simulink model "Modell_13_1_v2"  (R2018a)
settings: Solver=VariableStepAuto  StartTime=0.0  StopTime=10  MaxStep=0.001  RelTol=1e-3
InitFcn:
  | init_13_1_v2
values from neighbouring files (symbols this model uses):
  a = 1    [init_13_1.m]    (also in init_13_1_v2.m; init_13_4.m)
  b = 1    [init.m]    (also in init_13_1.m; init_13_1_v2.m = 0.1111; init_13_4.m)
  c = 0.5    [init.m]    (also in init_13_1.m; init_13_1_v2.m = 0.8333; init_13_4.m = 1)
  grenze = 20    [init_13_1_v2.m]
  grenzeSalz = 30    [init_13_1_v2.m]
  kS = 1    [init_13_1_v2.m]    (also in init_13_4.m = 0.3)
  kT = 1    [init_13_1_v2.m]    (also in init_13_4.m)
  kw = 0.1    [init_13_1_v2.m]
  kwS = 0.35    [init_13_1_v2.m]
  S01 = 30    [init_13_1_v2.m]    (also in init_13_4.m = 1.7)
  S02 = 35    [init_13_1_v2.m]    (also in init_13_4.m = 0.5)
  S1 = 31.87    [init_13_1_v2.m]
  S2 = 33.13    [init_13_1_v2.m]
  T01 = 29    [init_13_1_v2.m]    (also in init_13_4.m = 1.9)
  T02 = 12    [init_13_1_v2.m]    (also in init_13_4.m = 0.8)
  T1 = 10.8    [init_13_1_v2.m]
  T2 = 9.2    [init_13_1_v2.m]
libraries: simulink x2
settings Model: Creator=Uni  LastModifiedBy=Uni

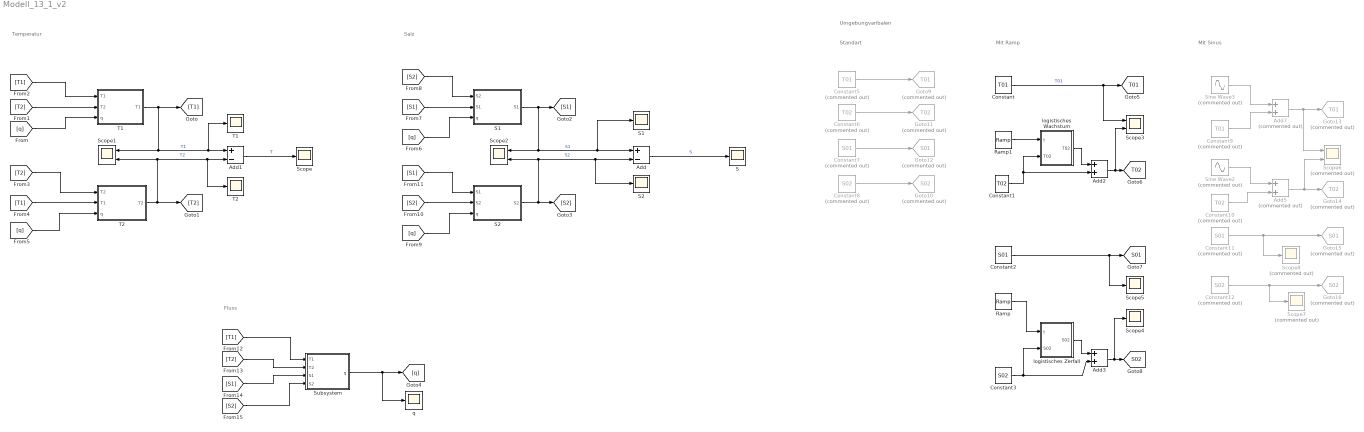
== system Modell_13_1_v2 ==
  note: Temperatur
  note: Salz
  note: Fluss
  note: Umgebungvaribalen
  note: Standart
  note: Mit Ramp
  note: Mit Sinus
  Add : Sum  Inputs=+-
  Add1 : Sum  Inputs=+-
  Add2 : Sum
  Add3 : Sum
  Add5 : Sum  Commented=on
  Add7 : Sum  Commented=on
  Constant : Constant  Value=T01
  Constant1 : Constant  Value=T02
  Constant10 : Constant  Commented=on  Value=T02
  Constant11 : Constant  Commented=on  Value=S01
  Constant12 : Constant  Commented=on  Value=S02
  Constant2 : Constant  Value=S01
  Constant3 : Constant  Value=S02
  Constant5 : Constant  Commented=on  Value=T01
  Constant6 : Constant  Commented=on  Value=T02
  Constant7 : Constant  Commented=on  Value=S01
  Constant8 : Constant  Commented=on  Value=S02
  Constant9 : Constant  Commented=on  Value=T01
  Goto10 : Goto  Commented=on  GotoTag=S02  TagVisibility=global
  Goto11 : Goto  Commented=on  GotoTag=T02  TagVisibility=global
  Goto12 : Goto  Commented=on  GotoTag=S01  TagVisibility=global
  Goto13 : Goto  Commented=on  GotoTag=T01  TagVisibility=global
  Goto14 : Goto  Commented=on  GotoTag=T02  TagVisibility=global
  Goto15 : Goto  Commented=on  GotoTag=S01  TagVisibility=global
  Goto16 : Goto  Commented=on  GotoTag=S02  TagVisibility=global
  Goto9 : Goto  Commented=on  GotoTag=T01  TagVisibility=global
  Ramp : simulink/Sources/Ramp  slope=1  start=0  InitialOutput=0
  Ramp1 : simulink/Sources/Ramp  slope=1  start=0  InitialOutput=0
  S : Scope
  S1 : Scope
  "S1 " : Subsystem
  S2 : Scope
  "S2 " : Subsystem
  Scope : Scope
  Scope1 : Scope  NumInputPorts=2
  Scope2 : Scope  NumInputPorts=2
  Scope3 : Scope  NumInputPorts=2
  Scope4 : Scope
  Scope5 : Scope
  Scope6 : Scope  Commented=on  NumInputPorts=2
  Scope7 : Scope  Commented=on
  Scope8 : Scope  Commented=on
  Sine Wave2 : Sin  Commented=on  Amplitude=7  Frequency=2*pi  Phase=pi/2  SampleTime=0
  Sine Wave3 : Sin  Commented=on  Amplitude=4  Frequency=2*pi  Phase=pi/2  SampleTime=0
  Subsystem : Subsystem
  T1 : Subsystem
  "T1 " : Scope
  T2 : Subsystem
  "T2 " : Scope
  logistisches Wachstum : Subsystem
  logistisches Zerfall : Subsystem
  q : Scope
  tag scope: S01=global, S02=global, T01=global, T02=global
  wires:
  [T1] -> T1/1("T1 ")
  [T2] -> T1/2("T2 ")
  [q] -> T1/3("q ")
  T1/1(T1) -> Scope1/1, "T1 "/1, Add1/1, [T1]  "T1"
  T2/1("T2 ") -> [T2], Scope1/2, "T2 "/1, Add1/2  "T2"
  [T2] -> T2/1("T2 ")
  [T1] -> T2/2(T1)
  [q] -> T2/3("q ")
  [S2] -> "S1 "/1(S2)
  [S1] -> "S1 "/2("S1 ")
  [q] -> "S1 "/3(q)
  "S1 "/1(S1) -> Scope2/1, S1/1, Add/1, [S1]  "S1"
  [q] -> "S2 "/3(q)
  "S2 "/1(S2) -> [S2], Scope2/2, S2/1, Add/2  "S2"
  [S2] -> "S2 "/2("S2 ")
  [S1] -> "S2 "/1("S1 ")
  [T1] -> Subsystem/1(T1)
  [T2] -> Subsystem/2(T2)
  [S1] -> Subsystem/3(S1)
  [S2] -> Subsystem/4(S2)
  Subsystem/1(q) -> q/1, [q]
  Add/1 -> S/1  "S"
  Add1/1 -> Scope/1  "T"
  Constant2/1 -> Scope5/1, [S01]
  Add3/1 -> Scope4/1, [S02]
  Constant5/1 -> Goto9/1
  Constant8/1 -> Goto10/1
  Constant6/1 -> Goto11/1
  Constant7/1 -> Goto12/1
  Add7/1 -> Scope6/1, Goto13/1
  Constant9/1 -> Add7/2
  Constant10/1 -> Add5/2
  Constant11/1 -> Scope8/1, Goto15/1
  Add5/1 -> Scope6/2, Goto14/1
  Sine Wave3/1 -> Add7/1
  Sine Wave2/1 -> Add5/1
  Constant12/1 -> Scope7/1, Goto16/1
  Constant/1 -> Scope3/1, [T01]  "T01"
  Ramp1/1 -> logistisches Wachstum/1(t)
  Constant1/1 -> Add2/2, logistisches Wachstum/2("T02 ")
  logistisches Wachstum/1(T02) -> Add2/1
  Add2/1 -> Scope3/2, [T02]
  logistisches Zerfall/1(S02) -> Add3/1
  Constant3/1 -> Add3/2, logistisches Zerfall/2("S02 ")
  Ramp/1 -> logistisches Zerfall/1(t)

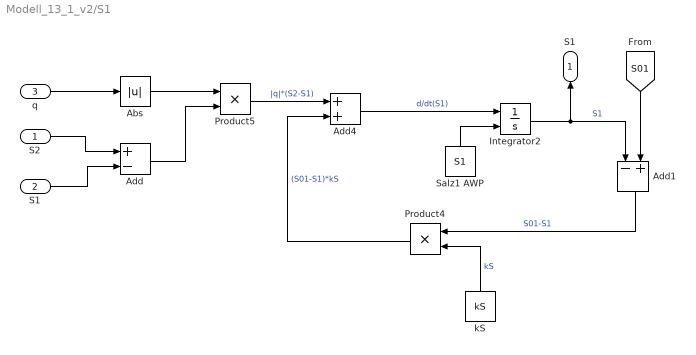
== system Modell_13_1_v2/S1  ==
  S2 : Inport
  "S1 " : Inport  Port=2
  q : Inport  Port=3
  Abs : Abs
  Add : Sum  Inputs=+-
  Add1 : Sum  Inputs=-+
  Add4 : Sum
  Integrator2 : Integrator  InitialConditionSource=external
  Product4 : Product
  Product5 : Product
  Salz1 AWP : Constant  Value=S1
  kS : Constant  Value=kS
  S1 : Outport
  wires:
  q/1 -> Abs/1
  Product4/1 -> Add4/2  "(S01-S1)*kS"
  Integrator2/1 -> Add1/1, S1/1  "S1"
  Add4/1 -> Integrator2/1  "d/dt(S1)"
  Product5/1 -> Add4/1  "|q|*(S2-S1)"
  Add/1 -> Product5/2
  Add1/1 -> Product4/1  "S01-S1"
  [S01] -> Add1/2
  S2/1 -> Add/1
  Salz1 AWP/1 -> Integrator2/2
  kS/1 -> Product4/2  "kS"
  "S1 "/1 -> Add/2
  Abs/1 -> Product5/1

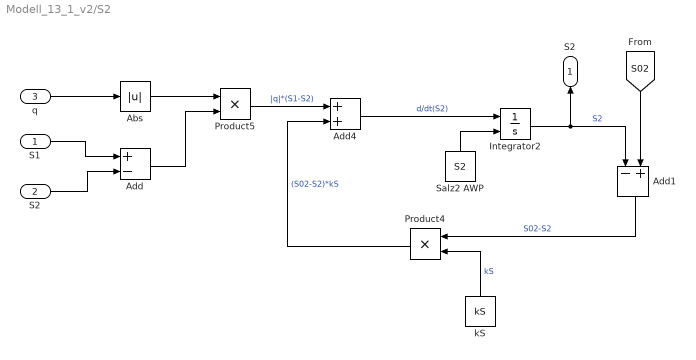
== system Modell_13_1_v2/S2  ==
  "S1 " : Inport
  "S2 " : Inport  Port=2
  q : Inport  Port=3
  Abs : Abs
  Add : Sum  Inputs=+-
  Add1 : Sum  Inputs=-+
  Add4 : Sum
  Integrator2 : Integrator  InitialConditionSource=external
  Product4 : Product
  Product5 : Product
  Salz2 AWP : Constant  Value=S2
  kS : Constant  Value=kS
  S2 : Outport
  wires:
  q/1 -> Abs/1
  Product4/1 -> Add4/2  "(S02-S2)*kS"
  Integrator2/1 -> Add1/1, S2/1  "S2"
  Add4/1 -> Integrator2/1  "d/dt(S2)"
  Product5/1 -> Add4/1  "|q|*(S1-S2)"
  Add/1 -> Product5/2
  Add1/1 -> Product4/1  "S02-S2"
  "S1 "/1 -> Add/1
  Salz2 AWP/1 -> Integrator2/2
  kS/1 -> Product4/2  "kS"
  "S2 "/1 -> Add/2
  Abs/1 -> Product5/1
  [S02] -> Add1/2

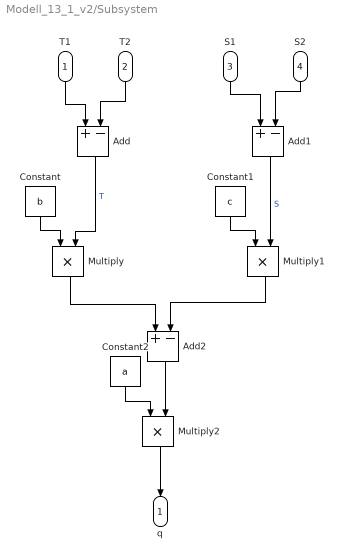
== system Modell_13_1_v2/Subsystem ==
  T1 : Inport
  T2 : Inport  Port=2
  S1 : Inport  Port=3
  S2 : Inport  Port=4
  Add : Sum  Inputs=+-
  Add1 : Sum  Inputs=+-
  Add2 : Sum  Inputs=+-
  Constant : Constant  Value=b
  Constant1 : Constant  Value=c
  Constant2 : Constant  Value=a
  Multiply : Product
  Multiply1 : Product
  Multiply2 : Product
  q : Outport
  wires:
  Add/1 -> Multiply/2  "T"
  Constant2/1 -> Multiply2/1
  Add1/1 -> Multiply1/2  "S"
  Constant1/1 -> Multiply1/1
  Multiply2/1 -> q/1
  Multiply/1 -> Add2/1
  Add2/1 -> Multiply2/2
  Multiply1/1 -> Add2/2
  Constant/1 -> Multiply/1
  T1/1 -> Add/1
  T2/1 -> Add/2
  S2/1 -> Add1/2
  S1/1 -> Add1/1

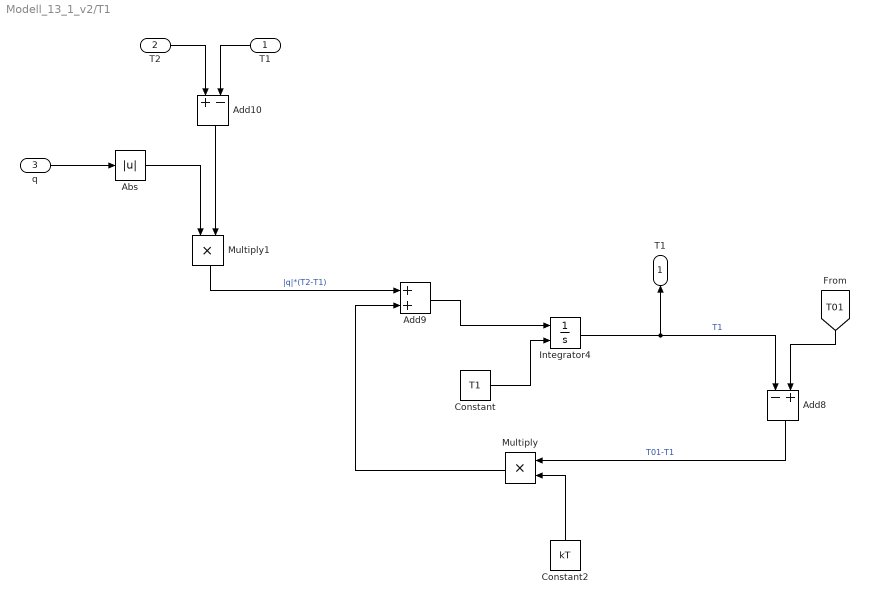
== system Modell_13_1_v2/T1 ==
  "T1 " : Inport
  "T2 " : Inport  Port=2
  "q " : Inport  Port=3
  Abs : Abs
  Add10 : Sum  Inputs=+-
  Add8 : Sum  Inputs=-+
  Add9 : Sum
  Constant : Constant  Value=T1
  Constant2 : Constant  Value=kT
  Integrator4 : Integrator  InitialConditionSource=external
  Multiply : Product
  Multiply1 : Product
  T1 : Outport
  wires:
  Add8/1 -> Multiply/1  "T01-T1"
  Multiply1/1 -> Add9/1  "|q|*(T2-T1)"
  Constant2/1 -> Multiply/2
  Add10/1 -> Multiply1/2
  "q "/1 -> Abs/1
  Constant/1 -> Integrator4/2
  Multiply/1 -> Add9/2
  Integrator4/1 -> Add8/1, T1/1  "T1"
  Add9/1 -> Integrator4/1
  [T01] -> Add8/2
  "T1 "/1 -> Add10/2
  "T2 "/1 -> Add10/1
  Abs/1 -> Multiply1/1

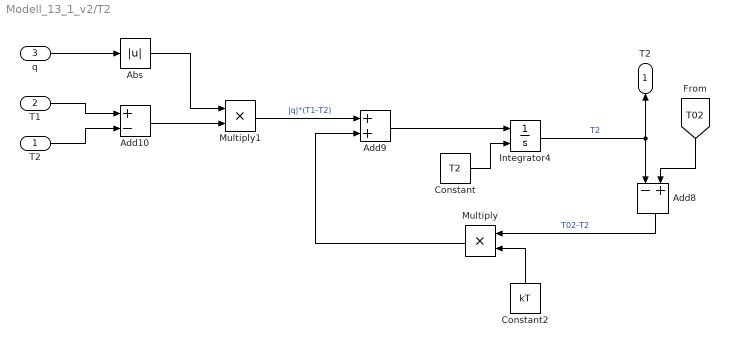
== system Modell_13_1_v2/T2 ==
  "T2 " : Inport
  T1 : Inport  Port=2
  "q " : Inport  Port=3
  Abs : Abs
  Add10 : Sum  Inputs=+-
  Add8 : Sum  Inputs=-+
  Add9 : Sum
  Constant : Constant  Value=T2
  Constant2 : Constant  Value=kT
  Integrator4 : Integrator  InitialConditionSource=external
  Multiply : Product
  Multiply1 : Product
  "T2 " : Outport
  wires:
  Add8/1 -> Multiply/1  "T02-T2"
  Multiply1/1 -> Add9/1  "|q|*(T1-T2)"
  Constant2/1 -> Multiply/2
  Add10/1 -> Multiply1/2
  "q "/1 -> Abs/1
  Constant/1 -> Integrator4/2
  Multiply/1 -> Add9/2
  Integrator4/1 -> Add8/1, "T2 "/1  "T2"
  Add9/1 -> Integrator4/1
  [T02] -> Add8/2
  "T2 "/1 -> Add10/2
  T1/1 -> Add10/1
  Abs/1 -> Multiply1/1

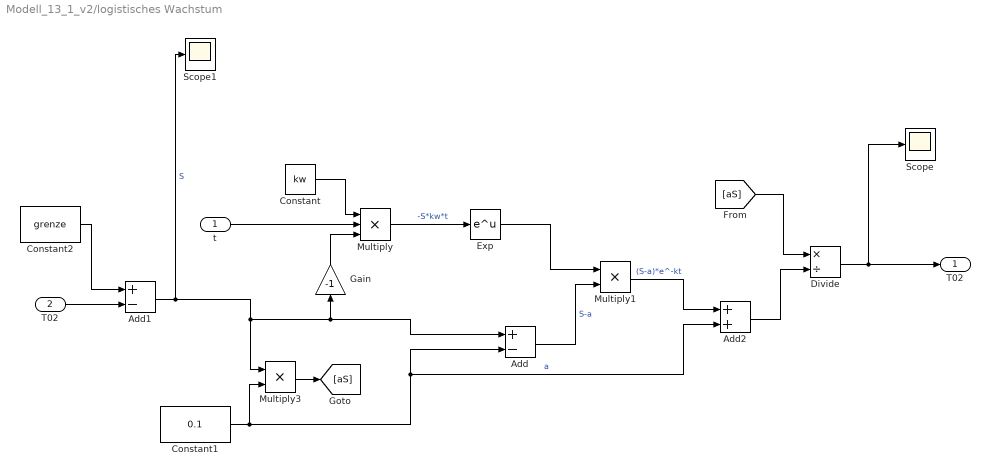
== system Modell_13_1_v2/logistisches Wachstum ==
  t : Inport
  "T02 " : Inport  Port=2
  Add : Sum  Inputs=+-
  Add1 : Sum  Inputs=+-
  Add2 : Sum
  Constant : Constant  Value=kw
  Constant1 : Constant  Value=0.1
  Constant2 : Constant  Value=grenze
  Divide : Product  Inputs=*/
  Exp : Math  SaturateOnIntegerOverflow=on
  Gain : Gain  Gain=-1
  Multiply : Product  Inputs=3
  Multiply1 : Product
  Multiply3 : Product
  Scope : Scope
  Scope1 : Scope
  T02 : Outport
  wires:
  Constant/1 -> Multiply/1
  t/1 -> Multiply/2
  Multiply/1 -> Exp/1  "-S*kw*t"
  Exp/1 -> Multiply1/1
  Multiply1/1 -> Add2/1  "(S-a)*e^-kt"
  Divide/1 -> Scope/1, T02/1
  Add/1 -> Multiply1/2  "S-a"
  Constant1/1 -> Multiply3/2, Add/2, Add2/2  "a"
  Add1/1 -> Scope1/1, Add/1, Gain/1, Multiply3/1  "S"
  Gain/1 -> Multiply/3
  Multiply3/1 -> [aS]
  Add2/1 -> Divide/2
  [aS] -> Divide/1
  Constant2/1 -> Add1/1
  "T02 "/1 -> Add1/2

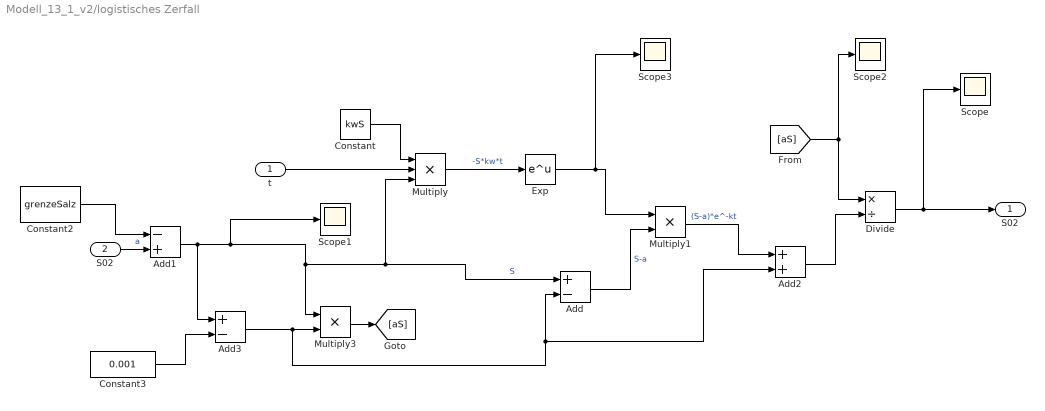
== system Modell_13_1_v2/logistisches Zerfall ==
  t : Inport
  "S02 " : Inport  Port=2
  Add : Sum  Inputs=+-
  Add1 : Sum  Inputs=-+
  Add2 : Sum
  Add3 : Sum  Inputs=+-
  Constant : Constant  Value=kwS
  Constant2 : Constant  Value=grenzeSalz
  Constant3 : Constant  Value=0.001
  Divide : Product  Inputs=*/
  Exp : Math  SaturateOnIntegerOverflow=on
  Multiply : Product  Inputs=3
  Multiply1 : Product
  Multiply3 : Product
  Scope{,1..3} (4 alike) : Scope
  S02 : Outport
  wires:
  Constant/1 -> Multiply/1
  t/1 -> Multiply/2
  Multiply/1 -> Exp/1  "-S*kw*t"
  Exp/1 -> Scope3/1, Multiply1/1
  Multiply1/1 -> Add2/1  "(S-a)*e^-kt"
  Divide/1 -> Scope/1, S02/1
  Add/1 -> Multiply1/2  "S-a"
  "S02 "/1 -> Add1/2  "a"
  Add1/1 -> Scope1/1, Multiply/3, Add/1, Multiply3/1, Add3/1  "S"
  Multiply3/1 -> [aS]
  Add2/1 -> Divide/2
  [aS] -> Scope2/1, Divide/1
  Constant2/1 -> Add1/1
  Add3/1 -> Add2/2, Add/2, Multiply3/2
  Constant3/1 -> Add3/2
